simulink model "Electric_powertrain"  (R2020b)
settings: Solver=FixedStepAuto  StartTime=0.0  StopTime=766  FixedStep=0.01  RelTol=1e-3
undefined symbols (not defined in the file): A, cd, eff_bat, eff_dt, eff_map, frr, g, i, m_t, mu, P_aux, P_max, r_d, rho, spd, torque
libraries: pid_lib x1
settings Model: Creator=yk_yo  LastModifiedBy=yk_yo

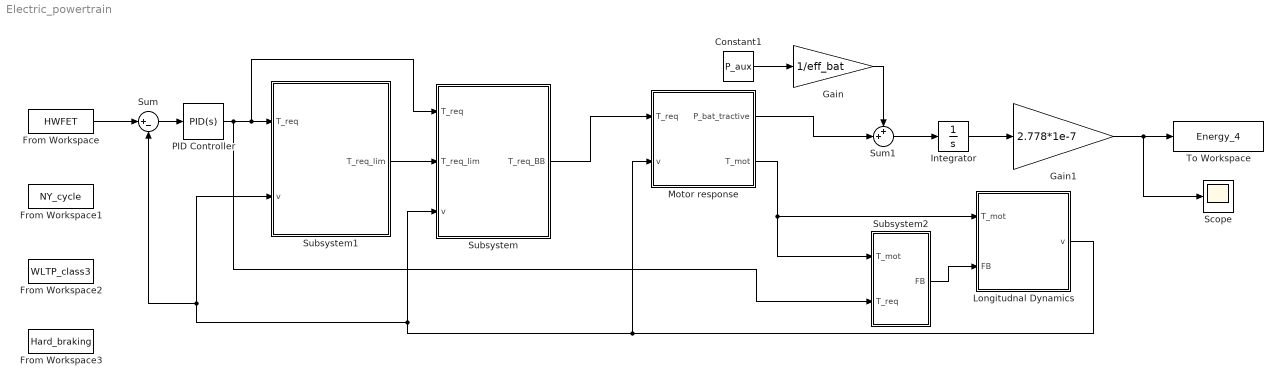
== system Electric_powertrain ==
  Constant1 : Constant  Value=P_aux
  From Workspace : FromWorkspace  VariableName=HWFET
  From Workspace1 : FromWorkspace  VariableName=NY_cycle
  From Workspace2 : FromWorkspace  VariableName=WLTP_class3
  From Workspace3 : FromWorkspace  VariableName=Hard_braking
  Gain : Gain  Gain=1/eff_bat
  Gain1 : Gain  Gain=2.778*1e-7
  Integrator : Integrator
  Longitudnal Dynamics : Subsystem
  Motor response : Subsystem
  PID Controller : pid_lib/PID Controller  Controller=PID  Form=Parallel  TimeDomain=Continuous-time  UseExternalTs=off  SampleTime=-1  IntegratorMethod=Forward Euler  FilterMethod=Forward Euler  ControllerParametersSource=internal  P=300  I=0  D=0  UseFilter=on  N=100  TunerSelectOption=Transfer Function Based (PID Tuner App)  InitialConditionSource=internal  InitialConditionForIntegrator=0  InitialConditionForFilter=0  DifferentiatorICPrevScaledInput=0  ExternalReset=none  TrackingMode=off  Kt=1  LimitOutput=on  SatLimitsSource=internal  UpperSaturationLimit=inf  LowerSaturationLimit=-(m_t*g*mu*r_d)/i  LinearizeAsGain=on  AntiWindupMode=none  Kb=1  POutMin=[]  POutMax=[]  IOutMin=[]  IOutMax=[]  DOutMin=[]  DOutMax=[]  NOutMin=[]  NOutMax=[]  SumOutMin=[]  SumOutMax=[]  SaturationOutMin=[]  SaturationOutMax=[]  PParamMin=[]  PParamMax=[]  IParamMin=[]  IParamMax=[]  DParamMin=[]  DParamMax=[]  NParamMin=[]  NParamMax=[]  KbParamMin=[]  KbParamMax=[]  KtParamMin=[]  KtParamMax=[]  KbOutMin=[]  KbOutMax=[]  KtOutMin=[]  KtOutMax=[]  IntegratorOutMin=[]  IntegratorOutMax=[]  FilterOutMin=[]  FilterOutMax=[]  SumI1OutMin=[]  SumI1OutMax=[]  SumI2OutMin=[]  SumI2OutMax=[]  SumI3OutMin=[]  SumI3OutMax=[]  SumI4OutMin=[]  SumI4OutMax=[]  SumDOutMin=[]  SumDOutMax=[]  DifferentiatorOutMin=[]  DifferentiatorOutMax=[]  FilterDiffOutCoefMin=[]  FilterDiffOutCoefMax=[]  ReciprocalOutMin=[]  ReciprocalOutMax=[]  SumDenOutMin=[]  SumDenOutMax=[]  SumNumOutMin=[]  SumNumOutMax=[]  DivideOutMin=[]  DivideOutMax=[]  UdiffTsProdOutMin=[]  UdiffTsProdOutMax=[]  NTsProdOutMin=[]  NTsProdOutMax=[]  UintegralTsProdOutMin=[]  UintegralTsProdOutMax=[]  UngainTsProdOutMin=[]  UngainTsProdOutMax=[]  IntegratorContinuousStateAttributes=''  IntegratorStateMustResolveToSignalObject=off  IntegratorRTWStateStorageClass=Auto  FilterContinuousStateAttributes=''  FilterStateMustResolveToSignalObject=off  FilterRTWStateStorageClass=Auto  ParallelPVariant=InternalParameters  IdealPVariant=Disabled  IVariant=InternalParameters  DVariant=InternalParameters  IntegratorVariant=Continuous  SatVariant=Enabled  AWVariant=Passthrough  PCopyVariant=Disabled  TRVariant=Disabled  FdbkBlocksVariant=Forward  IdealPFdbkVariant=Disabled  SatFdbkVariant=Disabled  DerivativeFilterVariant=ContFilter  NVariant=InternalParameters  NCopyVariant=Disabled  FilterICVariant=InternalICsFilter  IntegratorICVariant=InternalICs  ExternalResetVariant=Disabled  TRSumVariant=Passthrough  SumFdbkVariant=Disabled  SumVariant=Sum_PID  TsampFilterVariant=InternalTs  TsampNgainVariant=Passthrough  TsampIntegralVariant=Passthrough  ExternalSaturationOutDataTypeStr=Inherit: Same as second input
  Scope : Scope
  Subsystem : Subsystem
  Subsystem1 : Subsystem
  Subsystem2 : Subsystem
  Sum : Sum  Inputs=|+-
  Sum1 : Sum  Inputs=++|
  To Workspace : ToWorkspace  VariableName=Energy_4  SaveFormat=Timeseries  SampleTime=-1
  wires:
  Sum/1 -> PID Controller/1
  Motor response/1(P_bat_tractive) -> Sum1/2
  PID Controller/1 -> Subsystem2/2(T_req), Subsystem/1(T_req), Subsystem1/1(T_req)
  Motor response/2(T_mot) -> Subsystem2/1(T_mot), Longitudnal Dynamics/1(T_mot)
  Integrator/1 -> Gain1/1
  Constant1/1 -> Gain/1
  Sum1/1 -> Integrator/1
  Subsystem2/1(FB) -> Longitudnal Dynamics/2(FB)
  Subsystem1/1(T_req_lim) -> Subsystem/2(T_req_lim)
  Gain/1 -> Sum1/1
  Longitudnal Dynamics/1(v) -> Subsystem/3(v), Subsystem1/2(v), Sum/2, Motor response/2(v)
  Gain1/1 -> Scope/1, To Workspace/1
  Subsystem/1(T_req_BB) -> Motor response/1(T_req)
  From Workspace/1 -> Sum/1

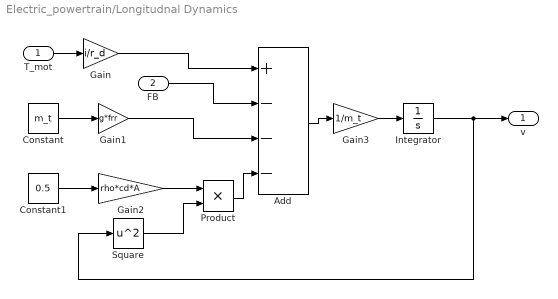
== system Electric_powertrain/Longitudnal Dynamics ==
  T_mot : Inport
  FB : Inport  Port=2
  Add : Sum  Inputs=+---
  Constant : Constant  Value=m_t
  Constant1 : Constant  Value=0.5
  Gain : Gain  Gain=i/r_d
  Gain1 : Gain  Gain=g*frr
  Gain2 : Gain  Gain=rho*cd*A
  Gain3 : Gain  Gain=1/m_t
  Integrator : Integrator
  Product : Product
  Square : Math  Operator=square  SaturateOnIntegerOverflow=on
  v : Outport
  wires:
  Constant/1 -> Gain1/1
  T_mot/1 -> Gain/1
  Square/1 -> Product/2
  Constant1/1 -> Gain2/1
  Gain2/1 -> Product/1
  Gain3/1 -> Integrator/1
  Integrator/1 -> Square/1, v/1
  Gain/1 -> Add/1
  Gain1/1 -> Add/3
  Product/1 -> Add/4
  FB/1 -> Add/2
  Add/1 -> Gain3/1

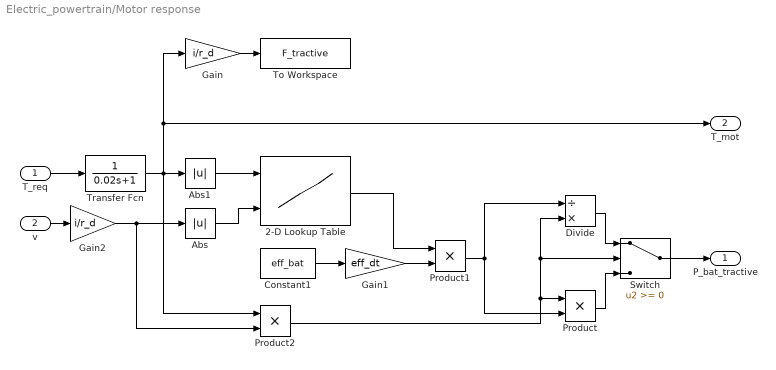
== system Electric_powertrain/Motor response ==
  T_req : Inport
  v : Inport  Port=2
  2-D Lookup Table : Lookup_n-D  BreakpointsForDimension1=[torque]  BreakpointsForDimension2=[spd]  Table=[eff_map]  InternalRulePriority=Speed  RndMeth=Simplest  InputSameDT=on
      settings: InputPortMap=u0,u1
  Abs : Abs
  Abs1 : Abs
  Constant1 : Constant  Value=eff_bat
  Divide : Product  Inputs=/*
  Gain : Gain  Gain=i/r_d
  Gain1 : Gain  Gain=eff_dt
  Gain2 : Gain  Gain=i/r_d
  Product : Product
  Product1 : Product
  Product2 : Product
  Switch : Switch
  To Workspace : ToWorkspace  VariableName=F_tractive  SaveFormat=Timeseries  SampleTime=-1
  Transfer Fcn : TransferFcn  Denominator=[0.02 1]
  P_bat_tractive : Outport
  T_mot : Outport  Port=2
  wires:
  Product/1 -> Switch/3
  v/1 -> Gain2/1
  2-D Lookup Table/1 -> Product1/1
  Divide/1 -> Switch/1
  Product1/1 -> Product/2, Divide/1
  Gain1/1 -> Product1/2
  Constant1/1 -> Gain1/1
  Abs/1 -> 2-D Lookup Table/2
  Abs1/1 -> 2-D Lookup Table/1
  Switch/1 -> P_bat_tractive/1
  Product2/1 -> Divide/2, Switch/2, Product/1
  Transfer Fcn/1 -> Gain/1, T_mot/1, Product2/1, Abs1/1
  T_req/1 -> Transfer Fcn/1
  Gain/1 -> To Workspace/1
  Gain2/1 -> Product2/2, Abs/1

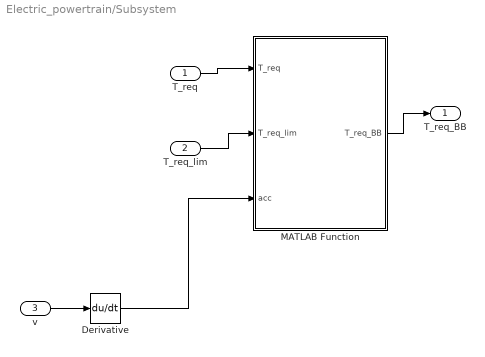
== system Electric_powertrain/Subsystem ==
  T_req : Inport
  T_req_lim : Inport  Port=2
  v : Inport  Port=3
  Derivative : Derivative
  MATLAB Function : MATLAB Function  TreatAsAtomicUnit=on
  T_req_BB : Outport
  wires:
  T_req/1 -> MATLAB Function/1(T_req)
  T_req_lim/1 -> MATLAB Function/2(T_req_lim)
  MATLAB Function/1(T_req_BB) -> T_req_BB/1
  v/1 -> Derivative/1
  Derivative/1 -> MATLAB Function/3(acc)

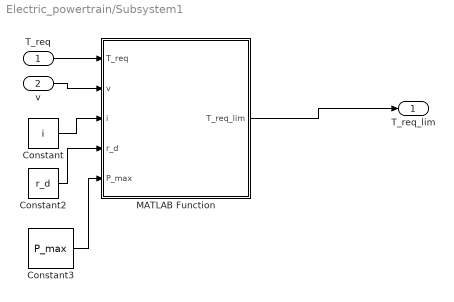
== system Electric_powertrain/Subsystem1 ==
  T_req : Inport
  v : Inport  Port=2
  Constant : Constant  Value=i
  Constant2 : Constant  Value=r_d
  Constant3 : Constant  Value=P_max
  MATLAB Function : MATLAB Function  TreatAsAtomicUnit=on
  T_req_lim : Outport
  wires:
  MATLAB Function/1(T_req_lim) -> T_req_lim/1
  Constant3/1 -> MATLAB Function/5(P_max)
  Constant/1 -> MATLAB Function/3(i)
  Constant2/1 -> MATLAB Function/4(r_d)
  v/1 -> MATLAB Function/2(v)
  T_req/1 -> MATLAB Function/1(T_req)

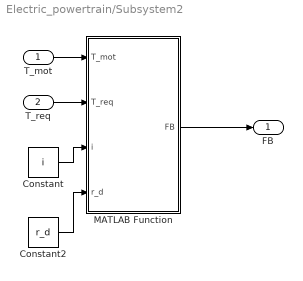
== system Electric_powertrain/Subsystem2 ==
  T_mot : Inport
  T_req : Inport  Port=2
  Constant : Constant  Value=i
  Constant2 : Constant  Value=r_d
  MATLAB Function : MATLAB Function  TreatAsAtomicUnit=on
  FB : Outport
  wires:
  MATLAB Function/1(FB) -> FB/1
  Constant/1 -> MATLAB Function/3(i)
  Constant2/1 -> MATLAB Function/4(r_d)
  T_req/1 -> MATLAB Function/2(T_req)
  T_mot/1 -> MATLAB Function/1(T_mot)

== matlab function Electric_powertrain/Subsystem/MATLAB Function ==
  data: T_req input; T_req_BB output; T_req_lim input; acc input
function T_req_BB = fcn(T_req,T_req_lim,acc)
g = 9.81;

if T_req < 0 && (acc) < 0
    
  if abs(acc)>0 && abs(acc)< 0.1*g
        T_req_BB = T_req_lim;
    elseif(abs(acc)> 0.1*g) && ( abs(acc) < (0.2*g))
     T_req_BB = 1.38 - ((3.8/g)*abs(acc));
    elseif  abs(acc) > 0.2*g
            T_req_BB = 0.62*T_req_lim;
    else 
           T_req_BB = T_req_lim; 
       
  end
else  
    T_req_BB = T_req_lim;
end

== matlab function Electric_powertrain/Subsystem1/MATLAB Function ==
  data: T_req input; T_req_lim output; v input; i input; r_d input; P_max input
function T_req_lim = fcn(T_req,v,i,r_d,P_max)
v1= v*3.6;
w_m = (v1*i)/r_d; %% angular velocity of motor
P = T_req*w_m; %% power calculation
 if T_req < 0 && v1 < 10 %% negative torque and 10kmph check
      T_req_lim = 0;
    else
        if T_req < -265 %% setting negative torque limit
            T_req_lim = -265;
        else
           if P < -1*P_max %% checking power limit for negative torque values
               T_req_lim = (-1*P_max)/w_m;
           else
               % T_req_lim = T_req; %% default torque
           
         
           
               if T_req>265  %% setting positive torque limit
                   T_req_lim = 265;
               else
                  if P > P_max  %% setting positive torque limit
                     T_req_lim = 140000/w_m;
                  else
                     T_req_lim = T_req; %% default torque
         
                  end
               end
           end
        end
 end
end

== matlab function Electric_powertrain/Subsystem2/MATLAB Function ==
  data: T_mot input; FB output; T_req input; i input; r_d input
function FB = fcn(T_mot,T_req,i,r_d)

if T_req<0 && T_mot>T_req
    FB = (T_mot-T_req)*(i/r_d);
else 
    FB = 0;
end
end
